simulink model "ballandgravityc"  (Simulink 7.1)
settings: Solver=ode45  StartTime=0.0  StopTime=10.0  RelTol=1e-3
undefined symbols (not defined in the file): g, k, m
settings Model: Creator=minakata  LastModifiedBy=minakata

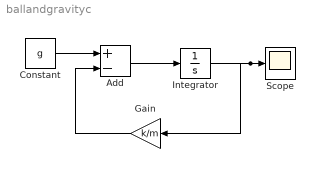
== system ballandgravityc ==
  Add : Sum  Inputs=+-  OutDataType=sfix(16)  OutScaling=2^-10
  Constant : Constant  Value=g  OutDataType=sfix(16)  OutScaling=2^0
  Gain : Gain  Orientation=left  Gain=k/m  ParameterDataType=sfix(16)  ParameterScaling=2^0  OutDataType=sfix(16)  OutScaling=2^0
  Integrator : Integrator
  Scope : Scope
  wires:
  Integrator/1 -> Scope/1, Gain/1
  Add/1 -> Integrator/1
  Constant/1 -> Add/1
  Gain/1 -> Add/2
